simulink model "E_Mod Simulink model"  (R2017a)
settings: Solver=ode45  StartTime=0.0  StopTime=10.0  RelTol=1e-3
undefined symbols (not defined in the file): param1
settings Model: Creator=patilomkarsudhir  LastModifiedBy=Win10
settings SolverCC: ZeroCrossAlgorithm=Adaptive
settings SFSimCC: SimUseLocalCustomCode=on
settings RTWCC: RTWUseLocalCustomCode=on

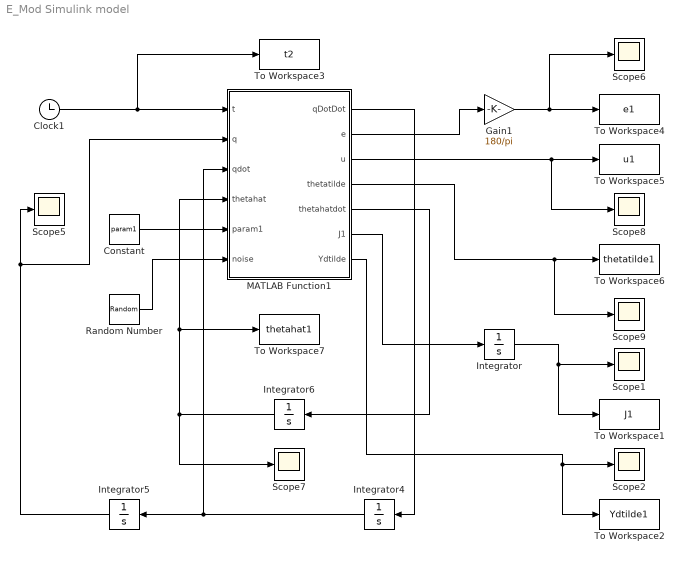
== system E_Mod Simulink model ==
  Clock1 : Clock
  Constant : Constant  Value=param1
  Gain1 : Gain  Gain=180/pi
  Integrator : Integrator
  Integrator4 : Integrator  InitialCondition=[0;0]
  Integrator5 : Integrator  InitialCondition=[-1;1]
  Integrator6 : Integrator  InitialCondition=zeros(7,1)
  MATLAB Function1 : MATLAB Function  TreatAsAtomicUnit=on
  Random Number : RandomNumber  Mean=[0;0;0;0]  Variance=(deg2rad(2)^2)*[1;1;1;1]  SampleTime=0.01  VectorParams1D=off
  Scope{1..2,5..9} (7 alike) : Scope
  To Workspace1 : ToWorkspace  VariableName=J1  SampleTime=-1
  To Workspace2 : ToWorkspace  VariableName=Ydtilde1  SampleTime=-1
  To Workspace3 : ToWorkspace  VariableName=t2  SampleTime=-1
  To Workspace4 : ToWorkspace  VariableName=e1  SampleTime=-1
  To Workspace5 : ToWorkspace  VariableName=u1  SampleTime=-1
  To Workspace6 : ToWorkspace  VariableName=thetatilde1  SampleTime=-1
  To Workspace7 : ToWorkspace  VariableName=thetahat1  SampleTime=-1
  wires:
  MATLAB Function1/5(thetahatdot) -> Integrator6/1
  MATLAB Function1/2(e) -> Gain1/1
  MATLAB Function1/4(thetatilde) -> Scope9/1, To Workspace6/1
  MATLAB Function1/1(qDotDot) -> Integrator4/1
  MATLAB Function1/3(u) -> To Workspace5/1, Scope8/1
  Integrator6/1 -> Scope7/1, To Workspace7/1, MATLAB Function1/4(thetahat)
  Integrator4/1 -> MATLAB Function1/3(qdot), Integrator5/1
  Clock1/1 -> To Workspace3/1, MATLAB Function1/1(t)
  Integrator5/1 -> Scope5/1, MATLAB Function1/2(q)
  Gain1/1 -> To Workspace4/1, Scope6/1
  Constant/1 -> MATLAB Function1/5(param1)
  MATLAB Function1/6(J1) -> Integrator/1
  Integrator/1 -> To Workspace1/1, Scope1/1
  MATLAB Function1/7(Ydtilde) -> To Workspace2/1, Scope2/1
  Random Number/1 -> MATLAB Function1/6(noise)

== matlab function E_Mod Simulink model/MATLAB Function1 ==
  data: t input; q input; qdot input; qDotDot output; e output; u output; thetatilde output; thetahatdot output; thetahat input; param1 input; J1 output; Ydtilde output; noise input
function [qDotDot,e,u,thetatilde,thetahatdot,J1,Ydtilde]  = fcn(t,q,qdot,thetahat,param1,noise)
% Declaring the desired q values and its differentials. 
qd=[cos(0.5*t);2*cos(t)];
qdDot=[-0.5*sin(0.5*t);-2*sin(t)]; 
qdDotDot=[-0.25*cos(0.5*t);-2*cos(t)]; 
qdDotDotDot=[0.125*sin(0.5*t);2*sin(t)]; 
qdDotDotDotDot=[0.0625*cos(0.5*t);2*cos(t)];
qd0=[1;2];
qdDot0=[0;0]; 


% Adding AWG noise to the q vector. Uncomment below 2 lines to check for AWG performance. 
% q=q+noise(1:2); 
% qdot=qdot+noise(3:4); 


q1=q(1); 
q2=q(2); 
q1dot=qdot(1); 
q2dot=qdot(2);
c2=cos(q2); 
s2=sin(q2); 
q10=-1; 
q20=1; 
q1dot0=0; 
q2dot0=3; 
c20=cos(q20);
s20=sin(q20);
c2d=cos(qd(2));
s2d=sin(qd(2));
c2d0=cos(qd0(2));
s2d0=sin(qd0(2));

% Calculating error in e
e=q-qd;
q0=[q10;q20];
qdot0=[q1dot0;q2dot0];

% Calculating tracking error
e10=q0-qd0;
e1dot0=qdot0-qdDot0;
edot=qdot-qdDot;
e1=e;
e1dot=edot;

% Declaring constant control gain alpha 
alpha=1;

% Calculating filtered tracking error
e2=e1dot+alpha*e1;
e20=e1dot0+alpha*e10;


% Calculating the regression matrix
Yd=[qdDotDot(1) qdDotDot(2) 2*c2d*qdDotDot(1)+c2d*qdDotDot(2)-s2d*qdDot(1)*qdDot(2)-s2d*(qdDot(1)+qdDot(2))*qdDot(2) qdDot(1) 0;
    0 qdDotDot(1)+qdDotDot(2) s2d*qdDot(1)^2+c2d*qdDotDot(2) 0 qdDot(2)];
Yd=[Yd eye(length(e))];


% Gamma=1;
% k=18.1506;

% Use below two lines for e-mod simulation.
Gamma=param1(1);
k=param1(2);
sigma=param1(3);



f=norm(thetahat)^2-400;
delf=2*thetahat;
prjscl=delf*delf'/norm(delf)^2;


thetahatdot=Gamma*Yd'*e2-sigma*norm(e1)*thetahat;
u=-Yd*thetahat-k*e2;


p1 = 3.473+0.5*sin(3*t);
p2 = 0.196+0.2*exp(-sin(t));
p3 = 0.242+0.1*cos(10*t);

fd1 = 5.3+2*exp(-0.1*t);
fd2 = 1.1+cos(5*t);
theta=[p1;p2;p3;fd1;fd2];
disturbance=[0.5*cos(0.5*t);sin(t)];
theta=[theta;disturbance];
thetatilde=theta-thetahat;
M = [p1+2*p3*cos(q(2)), p2+p3*cos(q(2)); p2+p3*cos(q(2)), p2];
Vm = [-p3*sin(q(2))*qdot(2), -p3*sin(q(2))*(qdot(1)+qdot(2)); p3*sin(q(2))*qdot(1), 0];
Fd = [fd1, 0; 0, fd2];

qDotDot = M\(u - Vm*qdot - Fd*qdot-disturbance);
J1=0.02*norm(u)^2+norm(e)^2;
Ydtilde=u+Yd*thetahat;
